simulink model "demoPure_teng4_sim2vrep_AdmitCtrl_Fext_VF"  (R2020a)
settings: Solver=FixedStepAuto  StartTime=0.0  StopTime=10  FixedStep=0.001  RelTol=1e-3
libraries: simulink_extras x2, simulink x1
settings Model: EnablePacing=on  Creator=jakub  LastModifiedBy=Teng
settings SolverCC: AutoInsertRateTranBlk=on
settings HardwareCC: ProdBitPerLong=64  ProdHWDeviceType=Intel->x86-64 (Linux 64)
settings SFSimCC: CustomCodeUndefinedFunction=UseInterfaceOnly

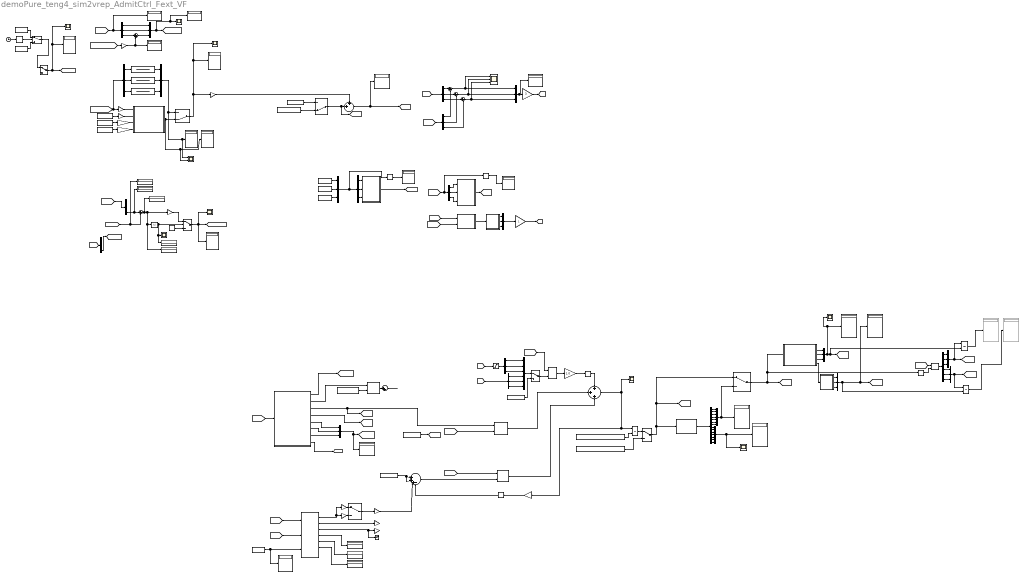
== system demoPure_teng4_sim2vrep_AdmitCtrl_Fext_VF ==
  note: VREP can be used only for visualization.
      | no VREP is also ok.
      |
      | in case of you are using VREP, load and use "teng4_panda.ttt" in VREP.
  note: Forward Kinematics of PANDA.
  note: get EE-related parameters,
      | (2) method-2, via derivative-Jacobian-integrator.
  note: get EE-related parameters,
      | (1) method-1, via Forward Kinematics
  note: here the two admittance model methods are exactly same.
  note: displacement caused by admittance model.
  note: initial ee
      | xyz [0.4682; 0; 0.6333]
      | rpy [3.138; 0.003525; -0.7857]
  note: 5
  note: results from both way (q_cmd or via VREP) should be the same.
      | But the 2nd way (via VREP) require a functional virtual robot in simulator (e.g. in VREP).
  note: verified!
      | almost same result from (1) and from (2). (very slightly difference.)
      | (1) left part, from q to Xee via forward kinematics;
      | (2) right part, from q to dq to dXee to Xee via derivative-integrator;
  note: initial x0 here should be the initial Xee position at the very beginning
  note: Jpinv: 7x6
  note: 7x6
  note: 7x1
  note: q_dot
  note: JT: 7X6
  note: J: 6X7
  note: Me=J*JT: 6X6
  note: NU: 7x7
  note: 10
  note: 7x6
  note: _ x
      | |\
      |   \
      |    \
  note: <------
      | y
  note: ^ z
      | |
      | |
      | |
  note: UDP Send.  joint velocity commands --> panda
      | ee velocity. 6x1. --> joint velocity 7x1
      |
      | remote ip: '127.0.0.1'
      | remote port: 39474
  note: define ee velocity,
      | based on desired/target x, y, z of ee.
  note: define ee rotation velocity,
      | based on desired/target rx, ry, rz of ee.
  note: set desired/target rx, ry, rz of ee.
  note: set desired/target x, y, z of ee.
  note: q_dot_NU
  note: to maxmize. using '+' gain.
  note: maximize rho.
      | rho, the manipulability along long axis of vME.
  note: teng4, rho. NULL-space optimization.
      | rho with direction u inside.
      | cost gradient.
  note: Jinv*X_dot_m
  note: q_dot_inv
  note: 7x1
  note: 7x1
  note: 7x1
  note: 7x7
  note: 7x1
  note: 7x1
  note: Vitual fixture
  note: external force from human, via Force sensor
  note: Virtual Fixture and Admittance control.
      | CoppeliaSim - Simulink Communication via S-function.
      | Version 1
      | Author : Teng Li.
      | teng4@ualberta.ca
      | University of Alberta
      | Edmonton, Canada.
      |
      | (updated date:2021-06-01)
  Abs1 : Abs
  Admittance model F : Subsystem
  Clock1 : Clock
  Constant1 : Constant  Value=[0;1;0]
  Constant20 : Constant  Value=0
  Constant21 : Constant  Value=pi
  Constant26 : Constant  Value=0
  Constant28 : Constant  Value=[1;1;1]
  Constant3 : Constant  Value=[0;0;0;0;0;0]  OutDataTypeStr=double
  Constant30 : Constant  Value=[1;1;1]
  Constant31 : Constant  Value=[1;1;1]
  Constant37 : Constant  Value=[0;0;0]
  Constant38 : Constant  Value=[0;0;-10]
  Constant5 : Constant  Value=pi/4
  Constant6 : Constant  Value=[1 1 1 1 1 1]
  Constant7 : Constant  Value=[0;0;0;0;0;0]  OutDataTypeStr=double
  Constant8 : Constant  Value=[0;0;0;0;0;0;0]  OutDataTypeStr=double
  Constant9 : Constant  Value=[0.4;0.1;0.3]
  CostFcnGradient4rho : MATLAB Function  TreatAsAtomicUnit=on
  Demux{1..2,8,10,12..17} (10 alike) : Demux  Outputs=3
  Demux3 : Demux  Outputs=6
  Demux9 : Demux  Outputs=14
  Derivative3 : Derivative
  Display{14,16,26,28,36..38,47,49..51,54..61,63..67} (24 alike) : Display
  Display44 : Display  Commented=on
  Display48 : Display  Commented=on
  Gain{1,4,12,14,16} (5 alike) : Gain
  Gain11 : Gain  Gain=-1
  Gain13 : Gain  Gain=80
  Gain15 : Gain  Gain=100
  Gain2 : Gain  Gain=1.0
  Gain3 : Gain  Gain=0.2
  Gain5 : Gain  Gain=0
  Gain6 : Gain  Gain=0
  Gain9 : Gain  Gain=0.01
  Integrator : Integrator  InitialConditionSource=external
  Integrator1 : Integrator  InitialConditionSource=external
  Integrator3 : Integrator  InitialConditionSource=external
  Interval Test : simulink/Logic and Bit Operations/Interval Test  IntervalClosedRight=on  uplimit=3  IntervalClosedLeft=on  lowlimit=2  OutDataTypeStr=boolean
  Joint q.now : Display
  Kp : Gain  Gain=3
  Kp.2 : Gain
  MATLAB Function12 : MATLAB Function  TreatAsAtomicUnit=on
  MATLAB Function7 : MATLAB Function  TreatAsAtomicUnit=on
  MATLAB Function9 : MATLAB Function  TreatAsAtomicUnit=on
  Manual Switch{,1,4,6,8} (5 alike) : ManualSwitch
  Manual Switch12 : ManualSwitch  CurrentSetting=0
  Manual Switch5 : ManualSwitch  CurrentSetting=0
  Matrix Multiply : Product  Multiplication=Matrix(*)
  Matrix Multiply2 : Product  Multiplication=Matrix(*)
  Memory : Memory
  Mux : Mux  Inputs=6
  Mux{1..2,6,8,12..15,17,19} (10 alike) : Mux  Inputs=3
  Mux11 : Mux  Inputs=7
  Mux9 : Mux  Inputs=7
  PandaForwardKinematics : MATLAB Function  TreatAsAtomicUnit=on
  Panda_fKine_q2xyz : MATLAB Function  TreatAsAtomicUnit=on
  PosError : Scope  NumInputPorts=3
  Product : Product  Multiplication=Matrix(*)
  Product2 : Product  Multiplication=Matrix(*)
  Product3 : Product  Multiplication=Matrix(*)
  Radians to Degrees2 : simulink_extras/Transformations/Radians to Degrees
  Radians to Degrees3 : simulink_extras/Transformations/Radians to Degrees
  Rate Limiter1 : RateLimiter  RisingSlewLimit=2.0  FallingSlewLimit=-2.0  SampleTimeMode=inherited
  S-Function2 : S-Function  FunctionName=teng4Sfcn_SIMtoVREP  SFunctionDeploymentMode=off  EnableBusSupport=off
  Saturation : Saturate  UpperLimit=0.1  LowerLimit=-0.1
  Scope4 : Scope  NumInputPorts=2
  Scope4_displacementBYadmittance : Scope
  Scope4_tau.now : Scope
  Scope5_F_vf : Scope
  Scope6 : Scope
  Scope7 : Scope
  Scope_F_ext : Scope
  Scope_Xee.pos : Scope
  Sum10 : Sum  Inputs=|++
  Sum11 : Sum  Inputs=|-+
  Sum12 : Sum  Inputs=++|
  Sum3 : Sum  Inputs=|+-
  Sum4 : Sum  Inputs=|+-
  Sum5 : Sum  Inputs=|+-
  Sum6 : Sum  Inputs=|++
  Sum7 : Sum  Inputs=||+++-
  Sum8 : Sum  Inputs=+++
  Switch : Switch  Criteria=u2 > Threshold  Threshold=0.0005
  Switch1 : Switch  Criteria=u2 > Threshold
  Terminator : Terminator
  Transfer Fcn10 : TransferFcn  Denominator=[1 80 100]
  Transfer Fcn11 : TransferFcn  Denominator=[1 80 100]
  Transfer Fcn12 : TransferFcn  Denominator=[1 80 100]
  VelocityOut1 : Scope
  in general2 : MATLAB Function  TreatAsAtomicUnit=on
  in general4 : MATLAB Function  TreatAsAtomicUnit=on
  initial pos in VREP : Constant  Value=[0.4682; 0; 0.6333]
  q0 initial pos in VREP : Constant  Value=[0.1223; -0.2672; -0.1022; -1.844; -0.02853; 1.574; -0.3199]
  q0 shapeOf7 : Constant  Value=[0; -0.266; 0; -1.84; 0; 1.569; 0.7873]
  tau.now : Display
  virtual fixture gain : Gain  Gain=50
  wires:
  Demux2/1 -> Mux/1
  Demux1/2 -> Mux/5
  Demux1/1 -> Mux/4
  Demux2/2 -> Mux/2
  Demux1/3 -> Mux/6
  Demux2/3 -> Mux/3
  [V_rot] -> Demux1/1
  [Jpinv] -> Matrix Multiply/1
  Demux15/1 -> Sum3/2
  Demux15/3 -> Sum4/2
  Sum3/1 -> Mux12/1, PosError/1
  Sum4/1 -> Mux12/3, PosError/3
  Demux16/1 -> Sum3/1
  Demux16/2 -> Sum5/1
  Demux16/3 -> Sum4/1
  [p_des] -> Demux16/1
  Demux15/2 -> Sum5/2
  Sum5/1 -> Mux12/2, PosError/2
  Gain2/1 -> Rate Limiter1/1
  Matrix Multiply/1 -> Gain2/1
  Kp/1 -> [V_cart]
  Mux12/1 -> Display14/1, Kp/1
  [Xee_pos] -> Demux15/1
  Manual Switch/1 -> Matrix Multiply/2
  Mux/1 -> Manual Switch/1
  Constant3/1 -> Manual Switch/2
  Kp.2/1 -> [V_rot]
  MATLAB Function9/1(R) -> [rot_des_so3]
  in general4/2(brad) -> Mux6/2
  [rot_des_so3] -> MATLAB Function12/1(R_des)
  in general4/1(arad) -> Mux6/1
  in general4/3(grad) -> Mux6/3
  MATLAB Function12/1(R_err) -> in general4/1(R)
  Mux6/1 -> Kp.2/1
  PandaForwardKinematics/2(JT) -> Product2/1
  PandaForwardKinematics/5(x_cart) -> Mux2/1
  Mux2/1 -> Display16/1, [X_pos_now]
  Constant6/1 -> Product2/2
  PandaForwardKinematics/8(Me_M) -> [Me_M]
  [Null_J] -> Product3/1
  PandaForwardKinematics/6(y_cart) -> Mux2/2
  [q_now] -> PandaForwardKinematics/1(q)
  PandaForwardKinematics/4(NU) -> [Null_J]
  PandaForwardKinematics/1(J) -> [J_panda]
  Product2/1 -> Sum6/1
  PandaForwardKinematics/7(z_cart) -> Mux2/3
  Sum6/1 -> ?
  Constant1/1 -> CostFcnGradient4rho/3(u), Display28/1
  [q_now] -> CostFcnGradient4rho/2(q)
  Product/1 -> Sum8/2
  Sum8/1 -> Gain9/1, Integrator/1, VelocityOut1/1
  Sum7/1 -> Product3/2
  Product3/1 -> Sum8/3
  Gain9/1 -> Memory/1
  [X_dot_6x1] -> Product/2
  PandaForwardKinematics/3(Jpinv) -> [Jpinv], Product/1
  Rate Limiter1/1 -> Sum8/1
  [J_panda] -> CostFcnGradient4rho/1(J)
  Constant7/1 -> [X_dot_6x1]
  CostFcnGradient4rho/2(drhoV_cf2) -> Gain3/1
  CostFcnGradient4rho/1(drho_cf1) -> Gain4/1, Gain11/1
  Memory/1 -> Sum7/4
  Gain11/1 -> Manual Switch4/2
  Gain4/1 -> Manual Switch4/1
  Manual Switch4/1 -> Gain5/1
  CostFcnGradient4rho/4(rho) -> Display36/1
  CostFcnGradient4rho/5(rhoV) -> Display37/1
  CostFcnGradient4rho/6(sigma) -> Display38/1
  CostFcnGradient4rho/3(dsigma_cf3) -> Gain6/1, Terminator/1
  Constant8/1 -> Sum7/2, Sum7/1
  Constant9/1 -> Manual Switch5/1
  Sum12/1 -> [p_des], Display26/1
  [J_panda] -> Matrix Multiply2/1
  Matrix Multiply2/1 -> Demux3/1
  Demux3/1 -> Mux1/1
  Demux3/2 -> Mux1/2
  Demux3/3 -> Mux1/3
  Demux3/4 -> Mux8/1
  Demux3/5 -> Mux8/2
  Demux3/6 -> Mux8/3
  Mux1/1 -> Integrator3/1, [dXee_pos]
  Mux8/1 -> Integrator1/1, [dXee_rpy]
  MATLAB Function7/1(R) -> [Xee_so3]
  [Xee_rpy] -> Radians to Degrees2/1, Demux8/1
  Demux8/1 -> MATLAB Function7/1(arad)
  Demux8/2 -> MATLAB Function7/2(brad)
  Demux8/3 -> MATLAB Function7/3(grad)
  [Xee_so3] -> MATLAB Function12/2(R_i)
  Demux9/1 -> Mux9/1
  Demux9/2 -> Mux9/2
  Demux9/3 -> Mux9/3
  Demux9/4 -> Mux9/4
  Demux9/5 -> Mux9/5
  Demux9/6 -> Mux9/6
  Demux9/7 -> Mux9/7
  Demux9/8 -> Mux11/1
  Demux9/9 -> Mux11/2
  Demux9/10 -> Mux11/3
  Demux9/11 -> Mux11/4
  Demux9/12 -> Mux11/5
  Demux9/13 -> Mux11/6
  Demux9/14 -> Mux11/7
  Manual Switch8/1 -> Panda_fKine_q2xyz/1(q), Derivative3/1, [q_now]
  Mux11/1 -> Scope4_tau.now/1, tau.now/1
  S-Function2/1 -> Demux9/1
  Panda_fKine_q2xyz/2(x_cart) -> Mux13/1
  Panda_fKine_q2xyz/3(y_cart) -> Mux13/2
  Panda_fKine_q2xyz/4(z_cart) -> Mux13/3
  Integrator3/1 -> Display48/1
  Radians to Degrees2/1 -> Display49/1
  Derivative3/1 -> Matrix Multiply2/2
  Manual Switch1/1 -> Manual Switch8/1, [q_cmd], S-Function2/1
  Mux13/1 -> Integrator3/2, [Xee_pos], Scope_Xee.pos/1, Display47/1
  in general2/2(brad) -> Mux15/2
  in general2/1(arad) -> Mux15/1
  Panda_fKine_q2xyz/5(X_so3) -> in general2/1(R)
  in general2/3(grad) -> Mux15/3
  Mux15/1 -> Integrator1/2, [Xee_rpy], Display50/1
  Integrator1/1 -> Display44/1
  Constant21/1 -> Mux14/1
  Constant20/1 -> Mux14/2
  Constant5/1 -> Mux14/3
  Demux10/1 -> MATLAB Function9/1(arad)
  Demux10/2 -> MATLAB Function9/2(brad)
  Demux10/3 -> MATLAB Function9/3(grad)
  Mux14/1 -> Radians to Degrees3/1, Demux10/1
  Radians to Degrees3/1 -> Display51/1
  Mux9/1 -> Manual Switch8/2, Joint q.now/1
  Gain5/1 -> Sum7/3
  Saturation/1 -> Demux2/1
  Manual Switch6/1 -> Display56/1, Scope_F_ext/1, [F_ext]
  Sum11/1 -> Display65/1, Abs1/1, Display59/1, virtual fixture gain/1
  Constant26/1 -> Switch/3
  [F_ext] -> Display63/1, Demux12/1
  virtual fixture gain/1 -> Switch/1
  Demux13/3 -> Sum11/1, Display57/1
  Constant31/1 -> Gain12/1
  [point_fixed] -> Sum11/2, Display58/1
  Constant28/1 -> Gain13/1
  Gain14/1 -> Admittance model F/1(F_Total)
  Gain12/1 -> Admittance model F/2(m)
  Abs1/1 -> Scope6/1, Display54/1, Switch/2
  Gain13/1 -> Admittance model F/3(c)
  [F_virtualFixture] -> Gain16/1
  Demux12/1 -> Mux19/1
  Constant30/1 -> Gain15/1
  Gain15/1 -> Admittance model F/4(k)
  Mux19/1 -> [F_total_admittance], Display61/1, Scope7/1
  Demux12/2 -> Mux19/2
  Demux12/3 -> Sum10/1
  Sum10/1 -> Mux19/3
  Gain16/1 -> Sum10/2, Display64/1
  Switch/1 -> Display60/1, Scope5_F_vf/1, [F_virtualFixture]
  [Xee_pos] -> Demux13/1
  Clock1/1 -> Interval Test/1
  Interval Test/1 -> Switch1/2
  Constant37/1 -> Switch1/3
  Constant38/1 -> Switch1/1
  Switch1/1 -> Manual Switch6/1
  initial pos in VREP/1 -> Manual Switch5/2
  Manual Switch5/1 -> [p1_fixed], Sum12/2
  Manual Switch12/1 -> Scope4_displacementBYadmittance/1, Display55/1, Gain1/1
  [F_total_admittance] -> Gain14/1, Demux14/1
  Transfer Fcn10/1 -> Mux17/1
  Transfer Fcn11/1 -> Mux17/2
  Transfer Fcn12/1 -> Mux17/3
  Demux14/3 -> Transfer Fcn12/1
  Demux14/2 -> Transfer Fcn11/1
  Demux14/1 -> Transfer Fcn10/1
  Mux17/1 -> Scope4/1, Display66/1, Manual Switch12/1
  Admittance model F/1(P_des_Cart) -> Manual Switch12/2, Scope4/2, Display67/1
  Demux17/3 -> [point_fixed]
  [V_cart] -> Saturation/1
  [p1_fixed] -> Demux17/1
  Gain1/1 -> Sum12/1
  q0 shapeOf7/1 -> Integrator/2
  Integrator/1 -> Manual Switch1/1
  q0 initial pos in VREP/1 -> Manual Switch1/2

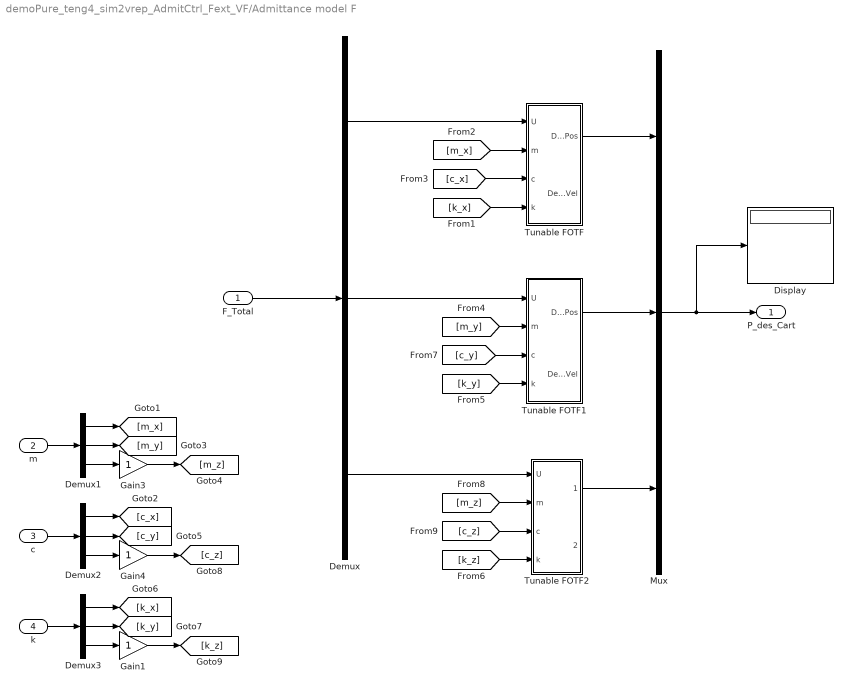
== system demoPure_teng4_sim2vrep_AdmitCtrl_Fext_VF/Admittance model F ==
  F_Total : Inport
  m : Inport  Port=2
  c : Inport  Port=3
  k : Inport  Port=4
  Demux{,1..3} (4 alike) : Demux  Outputs=3
  Display : Display
  Gain1 : Gain
  Gain3 : Gain
  Gain4 : Gain
  Mux : Mux  Inputs=3
  Tunable FOTF : Subsystem
  Tunable FOTF1 : Subsystem
  Tunable FOTF2 : Subsystem
  P_des_Cart : Outport  VectorParamsAs1DForOutWhenUnconnected=off
  wires:
  [m_y] -> Tunable FOTF1/2(m)
  Demux/1 -> Tunable FOTF/1(U)
  Tunable FOTF2/1(Des_Pos) -> Mux/3
  [m_z] -> Tunable FOTF2/2(m)
  Mux/1 -> Display/1, P_des_Cart/1
  [m_x] -> Tunable FOTF/2(m)
  Tunable FOTF/1(Des_Pos) -> Mux/1
  Demux/2 -> Tunable FOTF1/1(U)
  F_Total/1 -> Demux/1
  Tunable FOTF1/1(Des_Pos) -> Mux/2
  Demux/3 -> Tunable FOTF2/1(U)
  Demux2/2 -> [c_y]
  Demux1/2 -> [m_y]
  c/1 -> Demux2/1
  m/1 -> Demux1/1
  Demux2/1 -> [c_x]
  Demux1/1 -> [m_x]
  Demux2/3 -> Gain4/1
  Gain3/1 -> [m_z]
  Demux1/3 -> Gain3/1
  Gain4/1 -> [c_z]
  Gain1/1 -> [k_z]
  Demux3/3 -> Gain1/1
  k/1 -> Demux3/1
  Demux3/2 -> [k_y]
  Demux3/1 -> [k_x]
  [k_z] -> Tunable FOTF2/4(k)
  [c_z] -> Tunable FOTF2/3(c)
  [c_y] -> Tunable FOTF1/3(c)
  [k_y] -> Tunable FOTF1/4(k)
  [c_x] -> Tunable FOTF/3(c)
  [k_x] -> Tunable FOTF/4(k)

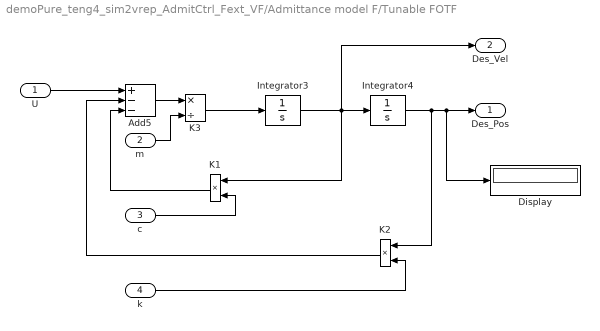
== system demoPure_teng4_sim2vrep_AdmitCtrl_Fext_VF/Admittance model F/Tunable FOTF ==
  U : Inport
  m : Inport  Port=2
  c : Inport  Port=3
  k : Inport  Port=4
  Add5 : Sum  Inputs=+--
  Display : Display
  Integrator3 : Integrator
  Integrator4 : Integrator
  K1 : Product  Inputs=**
  K2 : Product  Inputs=**
  K3 : Product  Inputs=*/
  Des_Pos : Outport  VectorParamsAs1DForOutWhenUnconnected=off
  Des_Vel : Outport  Port=2  VectorParamsAs1DForOutWhenUnconnected=off
  wires:
  U/1 -> Add5/1
  K3/1 -> Integrator3/1
  Add5/1 -> K3/1
  m/1 -> K3/2
  k/1 -> K2/2
  c/1 -> K1/2
  Integrator3/1 -> Integrator4/1, Des_Vel/1, K1/1
  Integrator4/1 -> K2/1, Display/1, Des_Pos/1
  K1/1 -> Add5/3
  K2/1 -> Add5/2

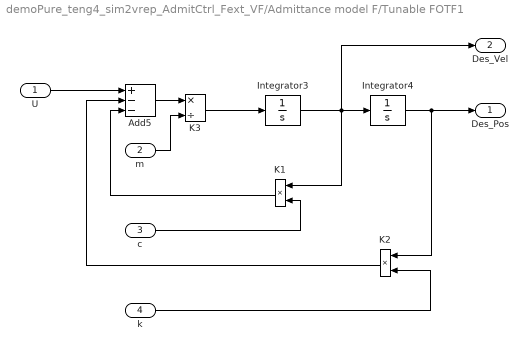
== system demoPure_teng4_sim2vrep_AdmitCtrl_Fext_VF/Admittance model F/Tunable FOTF1 ==
  U : Inport
  m : Inport  Port=2
  c : Inport  Port=3
  k : Inport  Port=4
  Add5 : Sum  Inputs=+--
  Integrator3 : Integrator
  Integrator4 : Integrator
  K1 : Product  Inputs=**
  K2 : Product  Inputs=**
  K3 : Product  Inputs=*/
  Des_Pos : Outport  VectorParamsAs1DForOutWhenUnconnected=off
  Des_Vel : Outport  Port=2  VectorParamsAs1DForOutWhenUnconnected=off
  wires:
  K3/1 -> Integrator3/1
  m/1 -> K3/2
  c/1 -> K1/2
  U/1 -> Add5/1
  k/1 -> K2/2
  Add5/1 -> K3/1
  Integrator3/1 -> Integrator4/1, Des_Vel/1, K1/1
  Integrator4/1 -> K2/1, Des_Pos/1
  K1/1 -> Add5/3
  K2/1 -> Add5/2

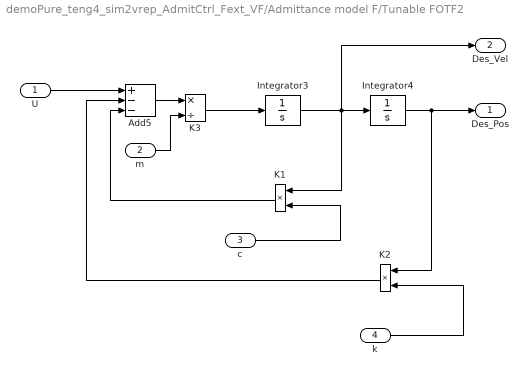
== system demoPure_teng4_sim2vrep_AdmitCtrl_Fext_VF/Admittance model F/Tunable FOTF2 ==
  U : Inport
  m : Inport  Port=2
  c : Inport  Port=3
  k : Inport  Port=4
  Add5 : Sum  Inputs=+--
  Integrator3 : Integrator
  Integrator4 : Integrator
  K1 : Product  Inputs=**
  K2 : Product  Inputs=**
  K3 : Product  Inputs=*/
  Des_Pos : Outport  VectorParamsAs1DForOutWhenUnconnected=off
  Des_Vel : Outport  Port=2  VectorParamsAs1DForOutWhenUnconnected=off
  wires:
  K3/1 -> Integrator3/1
  m/1 -> K3/2
  c/1 -> K1/2
  U/1 -> Add5/1
  k/1 -> K2/2
  Add5/1 -> K3/1
  Integrator3/1 -> Integrator4/1, Des_Vel/1, K1/1
  Integrator4/1 -> K2/1, Des_Pos/1
  K1/1 -> Add5/3
  K2/1 -> Add5/2

== matlab function demoPure_teng4_sim2vrep_AdmitCtrl_Fext_VF/MATLAB Function7 ==
  data: R output; arad input; brad input; grad input
function R  = rpy_to_so3(arad,brad,grad)
%#codegen
Rz = [cos(grad) -sin(grad) 0; sin(grad) cos(grad) 0; 0 0 1];
Ry = [cos(brad) 0 sin(brad); 0 1 0; -sin(brad) 0 cos(brad)];
Rx = [1 0 0; 0 cos(arad) -sin(arad); 0 sin(arad) cos(arad)];
R = Rz * Ry * Rx;

== matlab function demoPure_teng4_sim2vrep_AdmitCtrl_Fext_VF/Panda_fKine_q2xyz ==
  data: J output; q input; x_cart output; y_cart output; z_cart output; X_so3 output
function [J,x_cart,y_cart,z_cart,X_so3] = fcn_Panda_fkine_q2xyz(q)

q1 = q(1);
q2 = q(2);
q3 = q(3);
q4 = q(4);
q5 = q(5);
q6 = q(6);
q7 = q(7);

if 1 %Hongjun online method for Jacobian
    
% Define DH table & link transformation equation

%syms q1 q2 q3 q4 q5 q6 q7; %rotational angle for each link

% %DH table: [a d alpha theta], for Panda robot.
% dh_table = [0           0.333       0       q1
%             0           0          -pi/2    q2
%             0           0.316       pi/2    q3
%             0.0825      0           pi/2    q4
%            -0.0825      0.384      -pi/2    q5
%             0           0           pi/2    q6
%             0.088       0           pi/2    q7
%             0           0.107       0       0] %%the last row is for a Flange end-effector.

% %DH table: [a(m) alpha(rad) d(m) theta(rad)], for Panda robot.
% %DH table: [a alpha d theta]
dh_table = [0           0         0.333    q1
            0          -pi/2      0        q2
            0           pi/2      0.316    q3
            0.0825      pi/2      0        q4
           -0.0825     -pi/2      0.384    q5
            0           pi/2      0        q6
            0.088       pi/2      0        q7
            0           0         0.107    0 ]; %%the last row is for a Flange end-effector.


% %


% syms a alpha d theta;
% 
% % this T is using modified DH convention
% disp('--Here T is using modified DH convention.?')
% 
% T = [cos(theta)            -sin(theta)              0           a
%     sin(theta)*cos(alpha) cos(theta)*cos(alpha)   -sin(alpha) -sin(alpha)*d
%     sin(theta)*sin(alpha) cos(theta)*sin(alpha)    cos(alpha)  cos(alpha)*d
%     0                     0                        0           1]
% 
% T = [cos(dh_row(4))                -sin(dh_row(4))                   0               dh_row(1)
%      sin(dh_row(4))*cos(dh_row(2))  cos(dh_row(4))*cos(dh_row(2))   -sin(dh_row(2)) -sin(dh_row(2))*dh_row(3)
%      sin(dh_row(4))*sin(dh_row(2))  cos(dh_row(4))*sin(dh_row(2))    cos(dh_row(2))  cos(dh_row(2))*dh_row(3)
%      0                              0                                0               1]

%[a1, a2, a3, a4] = deal(1, 2, 3, 9)

% %
% deriving link transformations

% link 1
dh_row = dh_table(1,:); % specify a row of parameters for a certain link from DH table
T_0_1 = [cos(dh_row(4))                -sin(dh_row(4))                   0               dh_row(1)
     sin(dh_row(4))*cos(dh_row(2))  cos(dh_row(4))*cos(dh_row(2))   -sin(dh_row(2)) -sin(dh_row(2))*dh_row(3)
     sin(dh_row(4))*sin(dh_row(2))  cos(dh_row(4))*sin(dh_row(2))    cos(dh_row(2))  cos(dh_row(2))*dh_row(3)
     0                              0                                0               1];

% % link 2
dh_row = dh_table(2,:); % specify a row of parameters for a certain link from DH table
T_1_2 = [cos(dh_row(4))                -sin(dh_row(4))                   0               dh_row(1)
     sin(dh_row(4))*cos(dh_row(2))  cos(dh_row(4))*cos(dh_row(2))   -sin(dh_row(2)) -sin(dh_row(2))*dh_row(3)
     sin(dh_row(4))*sin(dh_row(2))  cos(dh_row(4))*sin(dh_row(2))    cos(dh_row(2))  cos(dh_row(2))*dh_row(3)
     0                              0                                0               1];

% % link 3
dh_row = dh_table(3,:); % specify a row of parameters for a certain link from DH table
T_2_3 = [cos(dh_row(4))                -sin(dh_row(4))                   0               dh_row(1)
     sin(dh_row(4))*cos(dh_row(2))  cos(dh_row(4))*cos(dh_row(2))   -sin(dh_row(2)) -sin(dh_row(2))*dh_row(3)
     sin(dh_row(4))*sin(dh_row(2))  cos(dh_row(4))*sin(dh_row(2))    cos(dh_row(2))  cos(dh_row(2))*dh_row(3)
     0                              0                                0               1];

% % link 4
dh_row = dh_table(4,:); % specify a row of parameters for a certain link from DH table
T_3_4 = [cos(dh_row(4))                -sin(dh_row(4))                   0               dh_row(1)
     sin(dh_row(4))*cos(dh_row(2))  cos(dh_row(4))*cos(dh_row(2))   -sin(dh_row(2)) -sin(dh_row(2))*dh_row(3)
     sin(dh_row(4))*sin(dh_row(2))  cos(dh_row(4))*sin(dh_row(2))    cos(dh_row(2))  cos(dh_row(2))*dh_row(3)
     0                              0                                0               1];

% % link 5
dh_row = dh_table(5,:); % specify a row of parameters for a certain link from DH table
T_4_5 = [cos(dh_row(4))                -sin(dh_row(4))                   0               dh_row(1)
     sin(dh_row(4))*cos(dh_row(2))  cos(dh_row(4))*cos(dh_row(2))   -sin(dh_row(2)) -sin(dh_row(2))*dh_row(3)
     sin(dh_row(4))*sin(dh_row(2))  cos(dh_row(4))*sin(dh_row(2))    cos(dh_row(2))  cos(dh_row(2))*dh_row(3)
     0                              0                                0               1];

% % link 6
dh_row = dh_table(6,:); % specify a row of parameters for a certain link from DH table
T_5_6 = [cos(dh_row(4))                -sin(dh_row(4))                   0               dh_row(1)
     sin(dh_row(4))*cos(dh_row(2))  cos(dh_row(4))*cos(dh_row(2))   -sin(dh_row(2)) -sin(dh_row(2))*dh_row(3)
     sin(dh_row(4))*sin(dh_row(2))  cos(dh_row(4))*sin(dh_row(2))    cos(dh_row(2))  cos(dh_row(2))*dh_row(3)
     0                              0                                0               1];

% % link 7
dh_row = dh_table(7,:); % specify a row of parameters for a certain link from DH table
T_6_7 = [cos(dh_row(4))                -sin(dh_row(4))                   0               dh_row(1)
     sin(dh_row(4))*cos(dh_row(2))  cos(dh_row(4))*cos(dh_row(2))   -sin(dh_row(2)) -sin(dh_row(2))*dh_row(3)
     sin(dh_row(4))*sin(dh_row(2))  cos(dh_row(4))*sin(dh_row(2))    cos(dh_row(2))  cos(dh_row(2))*dh_row(3)
     0                              0                                0               1];

% % link 8: end-effector, end point of link 7 with an extension
dh_row = dh_table(8,:); % specify a row of parameters for a certain link from DH table
T_7_8 = [cos(dh_row(4))                -sin(dh_row(4))                   0               dh_row(1)
     sin(dh_row(4))*cos(dh_row(2))  cos(dh_row(4))*cos(dh_row(2))   -sin(dh_row(2)) -sin(dh_row(2))*dh_row(3)
     sin(dh_row(4))*sin(dh_row(2))  cos(dh_row(4))*sin(dh_row(2))    cos(dh_row(2))  cos(dh_row(2))*dh_row(3)
     0                              0                                0               1];

%%%%%%%%%%%%%%%%%%%%%%%%%%%%%%%%%%%%%%%%
% % Hongjun online method for Jacobian
T_B_1 = T_0_1;
T_7_EE = T_7_8; 

% %
%Jacobian for the arm   
T_B_EE = T_B_1 * T_1_2 * T_2_3 * T_3_4 * T_4_5 * T_5_6 * T_6_7 * T_7_EE;


T_1_EE=T_1_2*T_2_3*T_3_4*T_4_5*T_5_6*T_6_7*T_7_EE;
J1x_all=cross(T_1_EE(1:3,4),T_1_EE(1:3,1));
J1x=J1x_all(3,1);
J1y_all=cross(T_1_EE(1:3,4),T_1_EE(1:3,2));
J1y=J1y_all(3,1); 
J1z_all=cross(T_1_EE(1:3,4),T_1_EE(1:3,3)); 
J1z=J1z_all(3,1); 
nz1=(T_1_EE(3,1));
oz1=(T_1_EE(3,2));
az1=(T_1_EE(3,3));

T_2_EE=T_2_3*T_3_4*T_4_5*T_5_6*T_6_7*T_7_EE;
J2x_all=cross(T_2_EE(1:3,4),T_2_EE(1:3,1));
J2x=(J2x_all(3,1));
J2y_all=cross(T_2_EE(1:3,4),T_2_EE(1:3,2));
J2y=(J2y_all(3,1));  
J2z_all=cross(T_2_EE(1:3,4),T_2_EE(1:3,3));
J2z=(J2z_all(3,1)); 
nz2=(T_2_EE(3,1));
oz2=(T_2_EE(3,2));
az2=(T_2_EE(3,3));

T_3_EE=T_3_4*T_4_5*T_5_6*T_6_7*T_7_EE;
J3x_all=cross(T_3_EE(1:3,4),T_3_EE(1:3,1));
J3x=(J3x_all(3,1));
J3y_all=cross(T_3_EE(1:3,4),T_3_EE(1:3,2));
J3y=(J3y_all(3,1)); 
J3z_all=cross(T_3_EE(1:3,4),T_3_EE(1:3,3));
J3z=(J3z_all(3,1));
nz3=(T_3_EE(3,1));
oz3=(T_3_EE(3,2));
az3=(T_3_EE(3,3));

T_4_EE=T_4_5*T_5_6*T_6_7*T_7_EE;
J4x_all=cross(T_4_EE(1:3,4),T_4_EE(1:3,1));
J4x=(J4x_all(3,1));
J4y_all=cross(T_4_EE(1:3,4),T_4_EE(1:3,2));
J4y=(J4y_all(3,1)); 
J4z_all=cross(T_4_EE(1:3,4),T_4_EE(1:3,3));
J4z=(J4z_all(3,1));
nz4=(T_4_EE(3,1));
oz4=(T_4_EE(3,2));
az4=(T_4_EE(3,3));

T_5_EE=T_5_6*T_6_7*T_7_EE;
J5x_all=cross(T_5_EE(1:3,4),T_5_EE(1:3,1));
J5x=(J5x_all(3,1));
J5y_all=cross(T_5_EE(1:3,4),T_5_EE(1:3,2));
J5y=(J5y_all(3,1)); 
J5z_all=cross(T_5_EE(1:3,4),T_5_EE(1:3,3));
J5z=(J5z_all(3,1));
nz5=(T_5_EE(3,1));
oz5=(T_5_EE(3,2));
az5=(T_5_EE(3,3));
 
T_6_EE=T_6_7*T_7_EE;
J6x_all=cross(T_6_EE(1:3,4),T_6_EE(1:3,1));
J6x=(J6x_all(3,1));
J6y_all=cross(T_6_EE(1:3,4),T_6_EE(1:3,2));
J6y=(J6y_all(3,1)) ;
J6z_all=cross(T_6_EE(1:3,4),T_6_EE(1:3,3));
J6z=(J6z_all(3,1));
nz6=(T_6_EE(3,1));
oz6=(T_6_EE(3,2));
az6=(T_6_EE(3,3));

J7x_all=cross(T_7_EE(1:3,4),T_7_EE(1:3,1));
J7x=(J7x_all(3,1));
J7y_all=cross(T_7_EE(1:3,4),T_7_EE(1:3,2));
J7y=(J7y_all(3,1)) ;
J7z_all=cross(T_7_EE(1:3,4),T_7_EE(1:3,3));
J7z=(J7z_all(3,1));
nz7=(T_7_EE(3,1));
oz7=(T_7_EE(3,2));
az7=(T_7_EE(3,3));


J_num = [T_B_EE(1:3,1:3),zeros(3,3);zeros(3,3),T_B_EE(1:3,1:3)]*... %Reference frame is the base frame
        [J1x J2x J3x J4x J5x J6x J7x;...
         J1y J2y J3y J4y J5y J6y J7y;...
         J1z J2z J3z J4z J5z J6z J7z;...
         nz1 nz2 nz3 nz4 nz5 nz6 nz7;...
         oz1 oz2 oz3 oz4 oz5 oz6 oz7;...
         az1 az2 az3 az4 az5 az6 az7];

end


J = J_num; %6x7
% JT=J'; %7x6
% Jpinv=pinv(J); %7x6
% %JinvM=M^(-1)*J'*(J*(M^(-1))*J')^-1;
% 
% NU=(eye(7)-J'*Jpinv'); %7x7
% %NUM=(eye(4)-J'*JinvM');


x_cart = T_B_EE(1,4);
y_cart = T_B_EE(2,4);
z_cart = T_B_EE(3,4);

% %JJT = J*J'; %2x4,4x2,=2x2
% %Me_M = [JJT(1,:),JJT(2,:)];
% JJT = J*J'; %6x7,7x6,=6x6
% %Me_M = [JJT(1,:),JJT(2,:),JJT(3,:),JJT(4,:),JJT(5,:),JJT(6,:)]; %6x6
% Me_M = [JJT(1,:);JJT(2,:);JJT(3,:);JJT(4,:);JJT(5,:);JJT(6,:)]; %6x6

X_so3 = T_B_EE(1:3,1:3);

== matlab function demoPure_teng4_sim2vrep_AdmitCtrl_Fext_VF/in general2 ==
  data: R input; arad output; brad output; grad output
function [arad,brad,grad] = so3_to_rpy(R)
sy = sqrt(R(3,2)^2 + R(3,3)^2);
if sy > eps
    % non singular
    arad = atan2(R(3,2),R(3,3));
    brad = atan2(-R(3,1),sy);
    grad = atan2(R(2,1),R(1,1));
else
    % singular
    arad = atan2(-R(2,3),R(2,2));
    brad = atan2(-R(3,1),sy);
    grad = 0;
end
end

== matlab function demoPure_teng4_sim2vrep_AdmitCtrl_Fext_VF/PandaForwardKinematics ==
  data: q input; J output; JT output; Jpinv output; NU output; x_cart output; y_cart output; z_cart output; Me_M output
function [J,JT,Jpinv,NU,x_cart,y_cart,z_cart,Me_M] = fcn_Panda_fkine(q)

q1 = q(1);
q2 = q(2);
q3 = q(3);
q4 = q(4);
q5 = q(5);
q6 = q(6);
q7 = q(7);

if 1 %Hongjun online method for Jacobian
    
% Define DH table & link transformation equation

%syms q1 q2 q3 q4 q5 q6 q7; %rotational angle for each link

% %DH table: [a d alpha theta], for Panda robot.
% dh_table = [0           0.333       0       q1
%             0           0          -pi/2    q2
%             0           0.316       pi/2    q3
%             0.0825      0           pi/2    q4
%            -0.0825      0.384      -pi/2    q5
%             0           0           pi/2    q6
%             0.088       0           pi/2    q7
%             0           0.107       0       0] %%the last row is for a Flange end-effector.

% %DH table: [a(m) alpha(rad) d(m) theta(rad)], for Panda robot.
% %DH table: [a alpha d theta]
dh_table = [0           0         0.333    q1
            0          -pi/2      0        q2
            0           pi/2      0.316    q3
            0.0825      pi/2      0        q4
           -0.0825     -pi/2      0.384    q5
            0           pi/2      0        q6
            0.088       pi/2      0        q7
            0           0         0.107    0 ]; %%the last row is for a Flange end-effector.


% %


% syms a alpha d theta;
% 
% % this T is using modified DH convention
% disp('--Here T is using modified DH convention.?')
% 
% T = [cos(theta)            -sin(theta)              0           a
%     sin(theta)*cos(alpha) cos(theta)*cos(alpha)   -sin(alpha) -sin(alpha)*d
%     sin(theta)*sin(alpha) cos(theta)*sin(alpha)    cos(alpha)  cos(alpha)*d
%     0                     0                        0           1]
% 
% T = [cos(dh_row(4))                -sin(dh_row(4))                   0               dh_row(1)
%      sin(dh_row(4))*cos(dh_row(2))  cos(dh_row(4))*cos(dh_row(2))   -sin(dh_row(2)) -sin(dh_row(2))*dh_row(3)
%      sin(dh_row(4))*sin(dh_row(2))  cos(dh_row(4))*sin(dh_row(2))    cos(dh_row(2))  cos(dh_row(2))*dh_row(3)
%      0                              0                                0               1]

%[a1, a2, a3, a4] = deal(1, 2, 3, 9)

% %
% deriving link transformations

% link 1
dh_row = dh_table(1,:); % specify a row of parameters for a certain link from DH table
T_0_1 = [cos(dh_row(4))                -sin(dh_row(4))                   0               dh_row(1)
     sin(dh_row(4))*cos(dh_row(2))  cos(dh_row(4))*cos(dh_row(2))   -sin(dh_row(2)) -sin(dh_row(2))*dh_row(3)
     sin(dh_row(4))*sin(dh_row(2))  cos(dh_row(4))*sin(dh_row(2))    cos(dh_row(2))  cos(dh_row(2))*dh_row(3)
     0                              0                                0               1];

% % link 2
dh_row = dh_table(2,:); % specify a row of parameters for a certain link from DH table
T_1_2 = [cos(dh_row(4))                -sin(dh_row(4))                   0               dh_row(1)
     sin(dh_row(4))*cos(dh_row(2))  cos(dh_row(4))*cos(dh_row(2))   -sin(dh_row(2)) -sin(dh_row(2))*dh_row(3)
     sin(dh_row(4))*sin(dh_row(2))  cos(dh_row(4))*sin(dh_row(2))    cos(dh_row(2))  cos(dh_row(2))*dh_row(3)
     0                              0                                0               1];

% % link 3
dh_row = dh_table(3,:); % specify a row of parameters for a certain link from DH table
T_2_3 = [cos(dh_row(4))                -sin(dh_row(4))                   0               dh_row(1)
     sin(dh_row(4))*cos(dh_row(2))  cos(dh_row(4))*cos(dh_row(2))   -sin(dh_row(2)) -sin(dh_row(2))*dh_row(3)
     sin(dh_row(4))*sin(dh_row(2))  cos(dh_row(4))*sin(dh_row(2))    cos(dh_row(2))  cos(dh_row(2))*dh_row(3)
     0                              0                                0               1];

% % link 4
dh_row = dh_table(4,:); % specify a row of parameters for a certain link from DH table
T_3_4 = [cos(dh_row(4))                -sin(dh_row(4))                   0               dh_row(1)
     sin(dh_row(4))*cos(dh_row(2))  cos(dh_row(4))*cos(dh_row(2))   -sin(dh_row(2)) -sin(dh_row(2))*dh_row(3)
     sin(dh_row(4))*sin(dh_row(2))  cos(dh_row(4))*sin(dh_row(2))    cos(dh_row(2))  cos(dh_row(2))*dh_row(3)
     0                              0                                0               1];

% % link 5
dh_row = dh_table(5,:); % specify a row of parameters for a certain link from DH table
T_4_5 = [cos(dh_row(4))                -sin(dh_row(4))                   0               dh_row(1)
     sin(dh_row(4))*cos(dh_row(2))  cos(dh_row(4))*cos(dh_row(2))   -sin(dh_row(2)) -sin(dh_row(2))*dh_row(3)
     sin(dh_row(4))*sin(dh_row(2))  cos(dh_row(4))*sin(dh_row(2))    cos(dh_row(2))  cos(dh_row(2))*dh_row(3)
     0                              0                                0               1];

% % link 6
dh_row = dh_table(6,:); % specify a row of parameters for a certain link from DH table
T_5_6 = [cos(dh_row(4))                -sin(dh_row(4))                   0               dh_row(1)
     sin(dh_row(4))*cos(dh_row(2))  cos(dh_row(4))*cos(dh_row(2))   -sin(dh_row(2)) -sin(dh_row(2))*dh_row(3)
     sin(dh_row(4))*sin(dh_row(2))  cos(dh_row(4))*sin(dh_row(2))    cos(dh_row(2))  cos(dh_row(2))*dh_row(3)
     0                              0                                0               1];

% % link 7
dh_row = dh_table(7,:); % specify a row of parameters for a certain link from DH table
T_6_7 = [cos(dh_row(4))                -sin(dh_row(4))                   0               dh_row(1)
     sin(dh_row(4))*cos(dh_row(2))  cos(dh_row(4))*cos(dh_row(2))   -sin(dh_row(2)) -sin(dh_row(2))*dh_row(3)
     sin(dh_row(4))*sin(dh_row(2))  cos(dh_row(4))*sin(dh_row(2))    cos(dh_row(2))  cos(dh_row(2))*dh_row(3)
     0                              0                                0               1];

% % link 8: end-effector, end point of link 7 with an extension
dh_row = dh_table(8,:); % specify a row of parameters for a certain link from DH table
T_7_8 = [cos(dh_row(4))                -sin(dh_row(4))                   0               dh_row(1)
     sin(dh_row(4))*cos(dh_row(2))  cos(dh_row(4))*cos(dh_row(2))   -sin(dh_row(2)) -sin(dh_row(2))*dh_row(3)
     sin(dh_row(4))*sin(dh_row(2))  cos(dh_row(4))*sin(dh_row(2))    cos(dh_row(2))  cos(dh_row(2))*dh_row(3)
     0                              0                                0               1];

%%%%%%%%%%%%%%%%%%%%%%%%%%%%%%%%%%%%%%%%
% % Hongjun online method for Jacobian
T_B_1 = T_0_1;
T_7_EE = T_7_8; 

% %
%Jacobian for the arm   
T_B_EE = T_B_1 * T_1_2 * T_2_3 * T_3_4 * T_4_5 * T_5_6 * T_6_7 * T_7_EE;
% T_B_EE=subs(T_B_EE,{q1 q2 q3,q4,q5, q6,q7},{ 0,1,0,0,0,0,0});
% T_B_EE=eval(T_B_EE)


T_1_EE=T_1_2*T_2_3*T_3_4*T_4_5*T_5_6*T_6_7*T_7_EE;
J1x_all=cross(T_1_EE(1:3,4),T_1_EE(1:3,1));
J1x=J1x_all(3,1);
J1y_all=cross(T_1_EE(1:3,4),T_1_EE(1:3,2));
J1y=J1y_all(3,1); 
J1z_all=cross(T_1_EE(1:3,4),T_1_EE(1:3,3)); 
J1z=J1z_all(3,1); 
% nz1=simplify(T_1_EE(3,1));
% oz1=simplify(T_1_EE(3,2));
% az1=simplify(T_1_EE(3,3));
nz1=(T_1_EE(3,1));
oz1=(T_1_EE(3,2));
az1=(T_1_EE(3,3));

T_2_EE=T_2_3*T_3_4*T_4_5*T_5_6*T_6_7*T_7_EE;
J2x_all=cross(T_2_EE(1:3,4),T_2_EE(1:3,1));
J2x=(J2x_all(3,1));
J2y_all=cross(T_2_EE(1:3,4),T_2_EE(1:3,2));
J2y=(J2y_all(3,1));  
J2z_all=cross(T_2_EE(1:3,4),T_2_EE(1:3,3));
J2z=(J2z_all(3,1)); 
nz2=(T_2_EE(3,1));
oz2=(T_2_EE(3,2));
az2=(T_2_EE(3,3));

T_3_EE=T_3_4*T_4_5*T_5_6*T_6_7*T_7_EE;
J3x_all=cross(T_3_EE(1:3,4),T_3_EE(1:3,1));
J3x=(J3x_all(3,1));
J3y_all=cross(T_3_EE(1:3,4),T_3_EE(1:3,2));
J3y=(J3y_all(3,1)); 
J3z_all=cross(T_3_EE(1:3,4),T_3_EE(1:3,3));
J3z=(J3z_all(3,1));
nz3=(T_3_EE(3,1));
oz3=(T_3_EE(3,2));
az3=(T_3_EE(3,3));

T_4_EE=T_4_5*T_5_6*T_6_7*T_7_EE;
J4x_all=cross(T_4_EE(1:3,4),T_4_EE(1:3,1));
J4x=(J4x_all(3,1));
J4y_all=cross(T_4_EE(1:3,4),T_4_EE(1:3,2));
J4y=(J4y_all(3,1)); 
J4z_all=cross(T_4_EE(1:3,4),T_4_EE(1:3,3));
J4z=(J4z_all(3,1));
nz4=(T_4_EE(3,1));
oz4=(T_4_EE(3,2));
az4=(T_4_EE(3,3));

T_5_EE=T_5_6*T_6_7*T_7_EE;
J5x_all=cross(T_5_EE(1:3,4),T_5_EE(1:3,1));
J5x=(J5x_all(3,1));
J5y_all=cross(T_5_EE(1:3,4),T_5_EE(1:3,2));
J5y=(J5y_all(3,1)); 
J5z_all=cross(T_5_EE(1:3,4),T_5_EE(1:3,3));
J5z=(J5z_all(3,1));
nz5=(T_5_EE(3,1));
oz5=(T_5_EE(3,2));
az5=(T_5_EE(3,3));
 
T_6_EE=T_6_7*T_7_EE;
J6x_all=cross(T_6_EE(1:3,4),T_6_EE(1:3,1));
J6x=(J6x_all(3,1));
J6y_all=cross(T_6_EE(1:3,4),T_6_EE(1:3,2));
J6y=(J6y_all(3,1)) ;
J6z_all=cross(T_6_EE(1:3,4),T_6_EE(1:3,3));
J6z=(J6z_all(3,1));
nz6=(T_6_EE(3,1));
oz6=(T_6_EE(3,2));
az6=(T_6_EE(3,3));

J7x_all=cross(T_7_EE(1:3,4),T_7_EE(1:3,1));
J7x=(J7x_all(3,1));
J7y_all=cross(T_7_EE(1:3,4),T_7_EE(1:3,2));
J7y=(J7y_all(3,1)) ;
J7z_all=cross(T_7_EE(1:3,4),T_7_EE(1:3,3));
J7z=(J7z_all(3,1));
nz7=(T_7_EE(3,1));
oz7=(T_7_EE(3,2));
az7=(T_7_EE(3,3));


J_num = [T_B_EE(1:3,1:3),zeros(3,3);zeros(3,3),T_B_EE(1:3,1:3)]*... %Reference frame is the base frame
        [J1x J2x J3x J4x J5x J6x J7x;...
         J1y J2y J3y J4y J5y J6y J7y;...
         J1z J2z J3z J4z J5z J6z J7z;...
         nz1 nz2 nz3 nz4 nz5 nz6 nz7;...
         oz1 oz2 oz3 oz4 oz5 oz6 oz7;...
         az1 az2 az3 az4 az5 az6 az7];

end


J = J_num; %6x7

JT=J'; %7x6


% Ib=11.09e-4;
% Ic=0.959e-4;
% Ia=0.486e-4;
% Id=7.11e-4;
% mc=0.0249;
% mb=0.2359;
% 
% lb=36.8e-3;
% % d3b=0
% ma=0.0202;
% 
% l3=0.0325;
% a1=0.06929+d(1)^2*.2; %a1=I1 + (d1^2*m1)/4 + d1^2*m2
% % a1=0.06929;
% a2=0.04217+d(1)*d(2)*.2; %a2=d1*d2*m2
% % a2=0.04217;
% a3=0.04416+(d(2)/2)^2*.2; %a3=I2+(d2^2*m2)/4 
% % a3=0.04416;


% M =[a1 + d(1)^2*ma + d(1)^2*mb + d(1)^2*mc, d(1)*d(3)*ma*cos(q(2) - q(1) + q(3)) + (d(1)*d(3)*mc*cos(q(2) - q(1) + q(3)))/2 + d(1)*lb*mb*cos(q(2) - q(1) + q(3)) + (d(1)*d(4)*ma*sin(q(2) - q(1) + q(4)))/2 - (a2*sin(q(1) - q(2)))/2 - d(1)*d(2)*ma*sin(q(1) - q(2)) - d(1)*d(2)*mb*sin(q(1) - q(2)) - d(1)*d(2)*mc*sin(q(1) - q(2)),                                                                     (d(1)*cos(q(2) - q(1) + q(3))*(2*d(3)*ma + d(3)*mc + 2*lb*mb))/2,                                                                  (d(1)*d(4)*ma*sin(q(2) - q(1) + q(4)))/2 - d(1)*l3*mc*sin(q(1) - q(4));
%  d(1)*d(3)*ma*cos(q(2) - q(1) + q(3)) + (d(1)*d(3)*mc*cos(q(2) - q(1) + q(3)))/2 + d(1)*lb*mb*cos(q(2) - q(1) + q(3)) + (d(1)*d(4)*ma*sin(q(2) - q(1) + q(4)))/2 - (a2*sin(q(1) - q(2)))/2 - d(1)*d(2)*ma*sin(q(1) - q(2)) - d(1)*d(2)*mb*sin(q(1) - q(2)) - d(1)*d(2)*mc*sin(q(1) - q(2)),    a3 + Ia + Ib + Ic + Id  + d(2)^2*ma + d(3)^2*ma + (d(4)^2*ma)/4 + d(2)^2*mb + d(2)^2*mc + (d(3)^2*mc)/4 + lb^2*mb + d(2)*d(4)*ma*cos(q(4)) - 2*d(2)*d(3)*ma*sin(q(3)) - d(2)*d(3)*mc*sin(q(3)) - 2*d(2)*lb*mb*sin(q(3)) - d(3)*d(4)*ma*sin(q(3) - q(4)), d(3)^2*ma + (d(3)^2*mc)/4 + lb^2*mb - d(2)*d(3)*ma*sin(q(3)) - (d(2)*d(3)*mc*sin(q(3)))/2 - d(2)*lb*mb*sin(q(3)) - (d(3)*d(4)*ma*sin(q(3) - q(4)))/2, (d(4)^2*ma)/4 - (d(3)*l3*mc*sin(q(2) + q(3) - q(4)))/2 + (d(2)*d(4)*ma*cos(q(4)))/2 + d(2)*l3*mc*cos(q(2) - q(4)) - (d(3)*d(4)*ma*sin(q(3) - q(4)))/2;
%  (d(1)*cos(q(2) - q(1) + q(3))*(2*d(3)*ma + d(3)*mc + 2*lb*mb))/2,                                                                                                      d(3)^2*ma + (d(3)^2*mc)/4 + lb^2*mb - d(2)*d(3)*ma*sin(q(3)) - (d(2)*d(3)*mc*sin(q(3)))/2 - d(2)*lb*mb*sin(q(3)) - (d(3)*d(4)*ma*sin(q(3) - q(4)))/2,                                                                                Ib + Ic + d(3)^2*ma + (d(3)^2*mc)/4 + lb^2*mb,                                                            - (d(3)*l3*mc*sin(q(2) + q(3) - q(4)))/2 - (d(3)*d(4)*ma*sin(q(3) - q(4)))/2;
%   (d(1)*d(4)*ma*sin(q(2) - q(1) + q(4)))/2 - d(1)*l3*mc*sin(q(1) - q(4)),                                                                                                       (d(4)^2*ma)/4 - (d(3)*l3*mc*sin(q(2) + q(3) - q(4)))/2 + (d(2)*d(4)*ma*cos(q(4)))/2 + d(2)*l3*mc*cos(q(2) - q(4)) - (d(3)*d(4)*ma*sin(q(3) - q(4)))/2,                                                             - (d(3)*l3*mc*sin(q(2) + q(3) - q(4)))/2 - (d(3)*d(4)*ma*sin(q(3) - q(4)))/2,                                                                                         (ma*d(4)^2)/4 + mc*l3^2 + Ia + Id];


Jpinv=pinv(J); %7x6
%JinvM=M^(-1)*J'*(J*(M^(-1))*J')^-1;

NU=(eye(7)-J'*Jpinv'); %7x7
%NUM=(eye(4)-J'*JinvM');


x_cart = T_B_EE(1,4);
y_cart = T_B_EE(2,4);
z_cart = T_B_EE(3,4);

%JJT = J*J'; %2x4,4x2,=2x2
%Me_M = [JJT(1,:),JJT(2,:)];
JJT = J*J'; %6x7,7x6,=6x6
%Me_M = [JJT(1,:),JJT(2,:),JJT(3,:),JJT(4,:),JJT(5,:),JJT(6,:)]; %6x6
Me_M = [JJT(1,:);JJT(2,:);JJT(3,:);JJT(4,:);JJT(5,:);JJT(6,:)]; %6x6

== matlab function demoPure_teng4_sim2vrep_AdmitCtrl_Fext_VF/in general4 ==
  data: R input; arad output; brad output; grad output
function [arad,brad,grad] = so3_to_rpy(R)
sy = sqrt(R(3,2)^2 + R(3,3)^2);
if sy > eps
    % non singular
    arad = atan2(R(3,2),R(3,3));
    brad = atan2(-R(3,1),sy);
    grad = atan2(R(2,1),R(1,1));
else
    % singular
    arad = atan2(-R(2,3),R(2,2));
    brad = atan2(-R(3,1),sy);
    grad = 0;
end
end

== matlab function demoPure_teng4_sim2vrep_AdmitCtrl_Fext_VF/MATLAB Function9 ==
  data: R output; arad input; brad input; grad input
function R  = rpy_to_so3(arad,brad,grad)
%#codegen
Rz = [cos(grad) -sin(grad) 0; sin(grad) cos(grad) 0; 0 0 1];
Ry = [cos(brad) 0 sin(brad); 0 1 0; -sin(brad) 0 cos(brad)];
Rx = [1 0 0; 0 cos(arad) -sin(arad); 0 sin(arad) cos(arad)];
R = Rz * Ry * Rx;

== matlab function demoPure_teng4_sim2vrep_AdmitCtrl_Fext_VF/MATLAB Function12 ==
  data: R_err output; R_des input; R_i input
function R_err  = R_err(R_des,R_i)
%#codegen
R_err = R_des*R_i';

== matlab function demoPure_teng4_sim2vrep_AdmitCtrl_Fext_VF/CostFcnGradient4rho ==
  data: J input; q input; drho_cf1 output; u input; drhoV_cf2 output; dsigma_cf3 output; rho output; rhoV output; sigma output; tt3 output
function [drho_cf1,drhoV_cf2,dsigma_cf3,rho,rhoV,sigma,tt3]  = fcn(J,q,u)

u = reshape(u,[3,1]); %ensure u direction is column vector by reshape.
J = reshape(J,[6,7]); %ensure u direction is column vector by reshape.
Jt = J(1:3,:); %J translational part, 3x7


%C = -sqrt(det(Me_c)) %eqn(22) in Robotica-2020
%effective manipulability, eqn(3) in Ali's IRAL-2019, also eqn(3) in Robotica-2020
%rho=(u'*(JJ')^(-1)*u)^(-1/2), rho is the major axis of vME.
%rho_temp = (u'*(J*J')^(-1)*u)^(-1/2); %rho for vME

q1=q(1);
q2=q(2);
q3=q(3);
q4=q(4);
q5=q(5);
q6=q(6);
q7=q(7);


if 1
% method-3, get dJ_q;
% test a new Jacobian derivative method
J_grad = teng4fcn_7dofPANDA_dJ_tensor(J);
J_grad_q1 = J_grad(:,:,1); %should be equal to dJ_q1
J_grad_q2 = J_grad(:,:,2); %should be equal to dJ_q2
J_grad_q3 = J_grad(:,:,3); %should be equal to dJ_q3
J_grad_q4 = J_grad(:,:,4); %should be equal to dJ_q4
J_grad_q5 = J_grad(:,:,5); %should be equal to dJ_q5
J_grad_q6 = J_grad(:,:,6); %should be equal to dJ_q6
J_grad_q7 = J_grad(:,:,7); %should be equal to dJ_q7
dJ_q1=J_grad_q1;
dJ_q2=J_grad_q2;
dJ_q3=J_grad_q3;
dJ_q4=J_grad_q4;
dJ_q5=J_grad_q5;
dJ_q6=J_grad_q6;
dJ_q7=J_grad_q7;

test3_grad=J_grad_q6;
tt3=test3_grad;
end

%dJ = dJ_q1*dq1+dJ_q2*dq2+dJ_q3*dq3+dJ_q4*dq4+dJ_q5*dq5+dJ_q6*dq6+dJ_q7*dq7;

dJ_q1 = reshape(dJ_q1,[6,7]); %reshape to ensure 6x7
dJ_q2 = reshape(dJ_q2,[6,7]); %reshape to ensure 6x7
dJ_q3 = reshape(dJ_q3,[6,7]); %reshape to ensure 6x7
dJ_q4 = reshape(dJ_q4,[6,7]); %reshape to ensure 6x7
dJ_q5 = reshape(dJ_q5,[6,7]); %reshape to ensure 6x7
dJ_q6 = reshape(dJ_q6,[6,7]); %reshape to ensure 6x7
dJ_q7 = reshape(dJ_q7,[6,7]); %reshape to ensure 6x7

dJt_q1 = dJ_q1(1:3,:); %3x7, only for translational Jacobian.
dJt_q2 = dJ_q2(1:3,:); %3x7, only for translational Jacobian.
dJt_q3 = dJ_q3(1:3,:); %3x7, only for translational Jacobian.
dJt_q4 = dJ_q4(1:3,:); %3x7, only for translational Jacobian.
dJt_q5 = dJ_q5(1:3,:); %3x7, only for translational Jacobian.
dJt_q6 = dJ_q6(1:3,:); %3x7, only for translational Jacobian.
dJt_q7 = dJ_q7(1:3,:); %3x7, only for translational Jacobian.

dJJT_q1 = dJ_q1*J'+J*dJ_q1'; %6x7,7x6; 6x7,7x6; 6x6
dJJT_q2 = dJ_q2*J'+J*dJ_q2'; %6x7,7x6; 6x7,7x6; 6x6
dJJT_q3 = dJ_q3*J'+J*dJ_q3'; %6x7,7x6; 6x7,7x6; 6x6
dJJT_q4 = dJ_q4*J'+J*dJ_q4'; %6x7,7x6; 6x7,7x6; 6x6
dJJT_q5 = dJ_q5*J'+J*dJ_q5'; %6x7,7x6; 6x7,7x6; 6x6
dJJT_q6 = dJ_q6*J'+J*dJ_q6'; %6x7,7x6; 6x7,7x6; 6x6
dJJT_q7 = dJ_q7*J'+J*dJ_q7'; %6x7,7x6; 6x7,7x6; 6x6

dJtJtT_q1 = dJt_q1*Jt'+Jt*dJt_q1'; %3x7,7x3; 3x7,7x3; 3x3
dJtJtT_q2 = dJt_q2*Jt'+Jt*dJt_q2'; %3x7,7x3; 3x7,7x3; 3x3
dJtJtT_q3 = dJt_q3*Jt'+Jt*dJt_q3'; %3x7,7x3; 3x7,7x3; 3x3
dJtJtT_q4 = dJt_q4*Jt'+Jt*dJt_q4'; %3x7,7x3; 3x7,7x3; 3x3
dJtJtT_q5 = dJt_q5*Jt'+Jt*dJt_q5'; %3x7,7x3; 3x7,7x3; 3x3
dJtJtT_q6 = dJt_q6*Jt'+Jt*dJt_q6'; %3x7,7x3; 3x7,7x3; 3x3
dJtJtT_q7 = dJt_q7*Jt'+Jt*dJt_q7'; %3x7,7x3; 3x7,7x3; 3x3

dsigma_q1=-0.5*u'*dJtJtT_q1*u/(u'*(Jt*Jt')*u)^1.5; %1x1
dsigma_q2=-0.5*u'*dJtJtT_q2*u/(u'*(Jt*Jt')*u)^1.5; %1x1
dsigma_q3=-0.5*u'*dJtJtT_q3*u/(u'*(Jt*Jt')*u)^1.5; %1x1
dsigma_q4=-0.5*u'*dJtJtT_q4*u/(u'*(Jt*Jt')*u)^1.5; %1x1
dsigma_q5=-0.5*u'*dJtJtT_q5*u/(u'*(Jt*Jt')*u)^1.5; %1x1
dsigma_q6=-0.5*u'*dJtJtT_q6*u/(u'*(Jt*Jt')*u)^1.5; %1x1
dsigma_q7=-0.5*u'*dJtJtT_q7*u/(u'*(Jt*Jt')*u)^1.5; %1x1

dsigma=[dsigma_q1,dsigma_q2,dsigma_q3,dsigma_q4,dsigma_q5,dsigma_q6,dsigma_q7]'; %7x1; force ME, sigma.
sigma=1/(u'*(Jt*Jt')*u)^0.5; %force ME, sigma.


drho_q1 = 0.5 * (u'*(Jt*Jt')^(-1)*u)^(-1.5) * (u'*(Jt*Jt')^(-2)*dJtJtT_q1*u); %1x1
drho_q2 = 0.5 * (u'*(Jt*Jt')^(-1)*u)^(-1.5) * (u'*(Jt*Jt')^(-2)*dJtJtT_q2*u); %1x1
drho_q3 = 0.5 * (u'*(Jt*Jt')^(-1)*u)^(-1.5) * (u'*(Jt*Jt')^(-2)*dJtJtT_q3*u); %1x1
drho_q4 = 0.5 * (u'*(Jt*Jt')^(-1)*u)^(-1.5) * (u'*(Jt*Jt')^(-2)*dJtJtT_q4*u); %1x1
drho_q5 = 0.5 * (u'*(Jt*Jt')^(-1)*u)^(-1.5) * (u'*(Jt*Jt')^(-2)*dJtJtT_q5*u); %1x1
drho_q6 = 0.5 * (u'*(Jt*Jt')^(-1)*u)^(-1.5) * (u'*(Jt*Jt')^(-2)*dJtJtT_q6*u); %1x1
drho_q7 = 0.5 * (u'*(Jt*Jt')^(-1)*u)^(-1.5) * (u'*(Jt*Jt')^(-2)*dJtJtT_q7*u); %1x1

%rho=(u'*(JJ')^(-1)*u)^(-1/2), rho is the major axis of vME.
drho=[drho_q1;drho_q2;drho_q3;drho_q4;drho_q5;drho_q6;drho_q7]; %7x1; velocity ME, rho.
rho = (u'*(Jt*Jt')^(-1)*u)^(-0.5); %rho, manipulability, vME


drhoV_q1 = 0.5 * (det(Jt*Jt'))^(-0.5) * trace((Jt*Jt')^(-1)*dJtJtT_q1); %1x1
drhoV_q2 = 0.5 * (det(Jt*Jt'))^(-0.5) * trace((Jt*Jt')^(-1)*dJtJtT_q2); %1x1
drhoV_q3 = 0.5 * (det(Jt*Jt'))^(-0.5) * trace((Jt*Jt')^(-1)*dJtJtT_q3); %1x1
drhoV_q4 = 0.5 * (det(Jt*Jt'))^(-0.5) * trace((Jt*Jt')^(-1)*dJtJtT_q4); %1x1
drhoV_q5 = 0.5 * (det(Jt*Jt'))^(-0.5) * trace((Jt*Jt')^(-1)*dJtJtT_q5); %1x1
drhoV_q6 = 0.5 * (det(Jt*Jt'))^(-0.5) * trace((Jt*Jt')^(-1)*dJtJtT_q6); %1x1
drhoV_q7 = 0.5 * (det(Jt*Jt'))^(-0.5) * trace((Jt*Jt')^(-1)*dJtJtT_q7); %1x1

%rhoV=sqrt(det(JJ')), rhoV is proportional to the volume V of vME
drhoV=[drhoV_q1;drhoV_q2;drhoV_q3;drhoV_q4;drhoV_q5;drhoV_q6;drhoV_q7]; %7x1; proportional to the velocity ME volume, rhoV.
rhoV = sqrt(det(Jt*Jt')); %rhoV, maximize it to avoid singularity.

drho_cf1 = drho; %7x1; velocity ME, maximizing for far away from singularity.
drhoV_cf2 = drhoV; %7x1; maximize it to avoid singularity
dsigma_cf3 = dsigma; %7x1; force ME, maximizing for close to singularity.
